simulink model "heli_q8"  (R2024b)
settings: Solver=ode1  StartTime=0.0  StopTime=inf  FixedStep=0.002  RelTol=1e-3  EnableMultiTasking=on
PostLoadFcn:
  | qc_set_target_type(getConfigSet(bdroot, 'QUARC Default Target Configuration'));
values from neighbouring files (symbols this model uses):
  A_d = 0    [kalman.m]
  B_d = 0    [kalman.m]
  C_d = 0    [kalman.m]
  Joystick_gain_x = 1    [kalman.m]
  Joystick_gain_y = -1    [kalman.m]
  Q_d = 0    [kalman.m]
  R_d = 0    [kalman.m]
  V_s0 = 0    [kalman.m]
undefined symbols (not defined in the file or in its folder): HIL, qc_get_step_size
libraries: quarc_library x4
settings Model: SimulationMode=external  ExtModeTrigDuration=5000  Creator=Rchan  LastModifiedBy=filip
settings SolverCC: AlgebraicLoopSolver=TrustRegion  PositivePriorityOrder=on
settings DataIOCC: LimitDataPoints=on  SaveFormat=Array  SignalLoggingSaveFormat=ModelDataLogs  ReturnWorkspaceOutputs=off
settings OptimizationCC: ExpressionDepthLimit=2147483647  InitFltsAndDblsToZero=on  LifeSpan=inf
settings DebuggingCC: SaveWithParameterizedLinksMsg=none  UnderspecifiedInitializationDetection=Classic  MergeDetectMultiDrivingBlocksExec=none  SolverPrmCheckMsg=warning  MultiTaskDSMMsg=warning  MultiTaskCondExecSysMsg=none  FcnCallInpInsideContextMsg=warning  UnconnectedInputMsg=warning  UnconnectedOutputMsg=warning  UnconnectedLineMsg=warning  AllowSymbolicDim=off  StateNameClashWarn=warning  SFUnexpectedBacktrackingDiag=warning  SFNoUnconditionalDefaultTransitionDiag=warning  SFExecutionAtInitializationDiag=none  ArithmeticOperatorsInVariantConditions=warning
settings HardwareCC: ProdBitPerPointer=32  ProdBitPerSizeT=32  ProdBitPerPtrDiffT=32  ProdLargestAtomicFloat=None  ProdIntDivRoundTo=Undefined  ProdEndianess=Unspecified  ProdWordSize=32  ProdHWDeviceType=32-bit Generic
settings ModelReferenceCC: EnableRefExpFcnMdlSchedulingChecks=on  PropagateSignalLabelsOutOfModel=off
settings SFSimCC: SimUseLocalCustomCode=off  CustomCodeUndefinedFunction=UseInterfaceOnly
settings RTWCC: Description=QUARC Win64 Target  SystemTargetFile=quarc_win64.tlc  TemplateMakefile=quarc_default_tmf  RTWUseLocalCustomCode=off  GPUComputeCapability=3.5
settings CodeAppCC: StateflowObjectComments=on
settings STFCustomTargetCC: TargetPreCompLibLocation=C:\PROGRA~3\QUARC\lib\2015b\win64\release  ConcurrentExecutionCompliant=on  CPPClassGenCompliant=on  GRTInterface=on  SystemTargetFile=quarc_win64.tlc
settings GRTTargetCC: TargetPreCompLibLocation=C:\PROGRA~3\QUARC\lib\2015b\win64\release  TargetLangStandard=C89/C90 (ANSI)  ParMdlRefBuildCompliant=off  CompOptLevelCompliant=off  CombineOutputUpdateFcns=off  MatFileLogging=off  GRTInterface=on  UseToolchainInfoCompliant=off  ExtMode=on  ExtModeMexFile=quarc_comm
settings ConfigComp: CovMetricSettings=dw  CovSaveCumulativeToWorkspaceVar=on  CovSaveSingleToWorkspaceVar=on  CovExternalEMLEnable=off  CovSFcnEnable=off

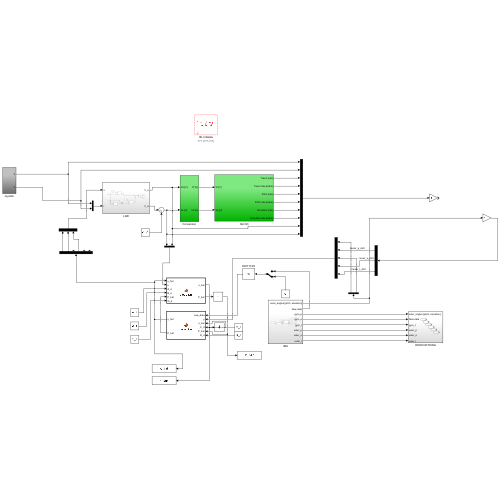
[thumbnail: Simulink's stored preview of the top-level diagram]
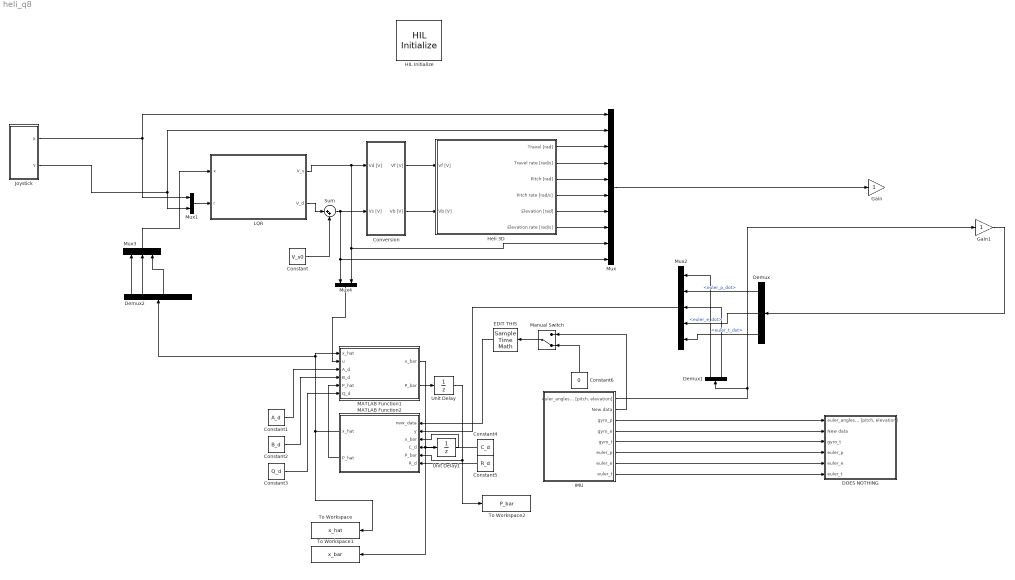
== system heli_q8 ==
  Constant : Constant  Value=V_s0
  Constant1 : Constant  Value=A_d
  Constant2 : Constant  Value=B_d
  Constant3 : Constant  Value=Q_d
  Constant4 : Constant  Value=C_d
  Constant5 : Constant  Value=R_d
  Constant6 : Constant  Value=0
  Conversion : Subsystem
  DOES NOTHING : Subsystem
  Demux : Demux  Outputs=3
  Demux1 : Demux  Outputs=2
  Demux2 : Demux  Outputs=6
  EDIT THIS : SampleTimeMath  TsampMathOp=Ts Only
  Gain : Gain
  Gain1 : Gain
  HIL Initialize : quarc_library/Data Acquisition/Generic/Configuration/HIL Initialize  Priority=-99  object_name=HIL-1  board_type=q8_usb  board_number=0  board_options=update_rate=normal;decimation=1  exclusive=off  active=off  hardware_clocks=[0:2]  clock_modes=[]  initial_clock_frequencies=[]  set_clock_params_at_start=off  set_clock_params_at_switch_in=off  set_clock_frequencies_at_start=off  set_clock_frequencies_at_switch_in=off  analog_input_channels=[0:7]  analog_input_maximums=10  analog_input_minimums=-10  set_analog_input_params_at_start=on  set_analog_input_params_at_switch_in=off  analog_output_channels=[0:7]  analog_output_maximums=10  analog_output_minimums=-10  initial_analog_outputs=[0]  final_analog_outputs=[0]  watchdog_analog_outputs=0  set_analog_output_params_at_start=on  set_analog_output_params_at_switch_in=off  set_analog_outputs_at_start=on  set_analog_outputs_at_switch_in=off  set_analog_outputs_at_terminate=on  set_analog_outputs_at_switch_out=off  set_analog_outputs_on_watchdog=off  digital_input_channels=[]  digital_output_channels=[]  digital_output_configuration=[]  initial_digital_outputs=[1]  final_digital_outputs=[1]  watchdog_digital_outputs=[1]  set_digital_output_params_at_start=off  set_digital_output_params_at_switch_in=off  set_digital_outputs_at_start=on  set_digital_outputs_at_switch_in=off  set_digital_outputs_at_terminate=on  set_digital_outputs_at_switch_out=off  set_digital_outputs_on_watchdog=off  encoder_channels=[0:7]  quadrature=[4]  encoder_filter_frequency=[]  initial_encoder_counts=[0]  set_encoder_params_at_start=on  set_encoder_params_at_switch_in=off  set_encoder_counts_at_start=on  set_encoder_counts_at_switch_in=off  pwm_channels=[0:7]  pwm_modes=0  pwm_frequency=99.532799999999995e6/4095  pwm_configuration=[0]  pwm_alignment=[0]  pwm_polarity=[1]  pwm_leading_deadband=[0]  pwm_trailing_deadband=[0]  initial_pwm_outputs=[0]  final_pwm_outputs=[0]  watchdog_pwm_outputs=[0]  set_pwm_params_at_start=on  set_pwm_params_at_switch_in=off  set_pwm_outputs_at_start=on  set_pwm_outputs_at_switch_in=off  set_pwm_outputs_at_terminate=on  set_pwm_outputs_at_switch_out=off  set_pwm_outputs_on_watchdog=off  other_output_channels=[]  initial_other_outputs=[]  final_other_outputs=[]  watchdog_other_outputs=[]  set_other_outputs_at_start=off  set_other_outputs_at_switch_in=off  set_other_outputs_at_terminate=off  set_other_outputs_at_switch_out=off  set_other_outputs_on_watchdog=off
  Heli 3D : Subsystem
  IMU : Subsystem
  Joystick : Subsystem
  LQR : Subsystem
  MATLAB Function1 : MATLAB Function  TreatAsAtomicUnit=on
  MATLAB Function2 : MATLAB Function  TreatAsAtomicUnit=on
  Manual Switch : ManualSwitch  CurrentSetting=0
  Mux : Mux  Inputs=10
  Mux1 : Mux  Inputs=2
  Mux2 : Mux  Inputs=5
  Mux3 : Mux  Inputs=3
  Mux4 : Mux  Inputs=2
  Sum : Sum  Inputs=|++
  To Workspace : ToWorkspace  VariableName=x_hat  SaveFormat=Timeseries  SampleTime=-1
  To Workspace1 : ToWorkspace  VariableName=x_bar  SaveFormat=Timeseries  SampleTime=-1
  To Workspace2 : ToWorkspace  VariableName=P_bar  SaveFormat=Timeseries  SampleTime=-1
  Unit Delay : UnitDelay  SampleTime=-1  HasFrameUpgradeWarning=on
  Unit Delay1 : UnitDelay  SampleTime=-1  HasFrameUpgradeWarning=on
  wires:
  Conversion/2(Vb [V]) -> Heli 3D/2(Vb [V])
  Conversion/1(Vf [V]) -> Heli 3D/1(Vf [V])
  Mux1/1 -> LQR/2(r)
  Joystick/1(X) -> Mux1/1, Mux/1
  Joystick/2(Y) -> Mux/2, Mux1/2
  Heli 3D/1(Travel [rad]) -> Mux/3
  Heli 3D/2(Travel rate [rad/s]) -> Mux/4
  Heli 3D/3(Pitch [rad]) -> Mux/5
  Heli 3D/4(Pitch rate [rad/s]) -> Mux/6
  Heli 3D/5(Elevation [rad]) -> Mux/7
  Heli 3D/6(Elevation rate [rad/s]) -> Mux/8
  LQR/1(V_s) -> Mux/9, Mux4/2, Conversion/1(Vd [V])
  LQR/2(V_d) -> Sum/1
  Constant/1 -> Sum/2
  Sum/1 -> Mux/10, Mux4/1, Conversion/2(Vs [V])
  Constant3/1 -> MATLAB Function1/6(Q_d)
  Constant2/1 -> MATLAB Function1/4(B_d)
  Constant1/1 -> MATLAB Function1/3(A_d)
  MATLAB Function2/2(P_hat) -> MATLAB Function1/5(P_hat)
  MATLAB Function2/1(x_hat) -> MATLAB Function1/1(x_hat), Demux2/1, To Workspace/1
  MATLAB Function1/1(x_bar) -> Unit Delay1/1, To Workspace1/1
  MATLAB Function1/2(P_bar) -> Unit Delay/1
  Unit Delay1/1 -> MATLAB Function2/3(x_bar)
  Unit Delay/1 -> To Workspace2/1, MATLAB Function2/5(P_bar)
  IMU/3(gyro_p) -> DOES NOTHING/1("euler_angles [pitch, elevation]")
  IMU/4(gyro_e) -> DOES NOTHING/2(New data)
  IMU/5(gyro_t) -> DOES NOTHING/3(gyro_t)
  IMU/6(euler_p) -> DOES NOTHING/4(euler_p)
  IMU/7(euler_e) -> DOES NOTHING/5(euler_e)
  IMU/8(euler_t) -> DOES NOTHING/6(euler_t)
  Mux/1 -> Gain/1
  IMU/1("euler_angles [pitch, elevation]") -> Demux1/1, Gain1/1
  Gain1/1 -> Demux/1
  Demux/3 -> Mux2/5  "<euler_t_dot>"
  Demux/2 -> Mux2/4  "<euler_e_dot>"
  Demux1/1 -> Mux2/1
  Demux1/2 -> Mux2/3
  Mux2/1 -> MATLAB Function2/2(y)
  Constant4/1 -> MATLAB Function2/4(C_d)
  Constant5/1 -> MATLAB Function2/6(R_d)
  Demux/1 -> Mux2/2  "<euler_p_dot>"
  EDIT THIS/1 -> MATLAB Function2/1(new_data)
  Manual Switch/1 -> EDIT THIS/1
  Constant6/1 -> Manual Switch/2
  IMU/2(New data) -> Manual Switch/1
  Demux2/1 -> Mux3/1
  Demux2/2 -> Mux3/2
  Demux2/4 -> Mux3/3
  Mux3/1 -> LQR/1(x)
  Mux4/1 -> MATLAB Function1/2(u)

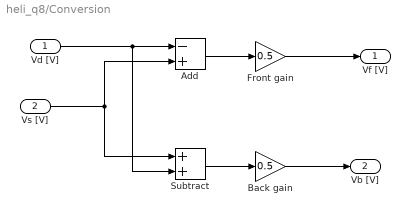
== system heli_q8/Conversion ==
  Vd [V] : Inport
  Vs [V] : Inport  Port=2
  Add : Sum  Inputs=-+
  Back gain : Gain  Gain=0.5
  Front gain : Gain  Gain=0.5
  Subtract : Sum
  Vf [V] : Outport
  Vb [V] : Outport  Port=2
  wires:
  Vd [V]/1 -> Subtract/2, Add/1
  Vs [V]/1 -> Subtract/1, Add/2
  Subtract/1 -> Back gain/1
  Back gain/1 -> Vb [V]/1
  Add/1 -> Front gain/1
  Front gain/1 -> Vf [V]/1

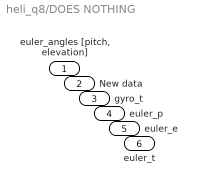
== system heli_q8/DOES NOTHING ==
  "euler_angles [pitch, elevation]" : Inport
  New data : Inport  Port=2
  gyro_t : Inport  Port=3
  euler_p : Inport  Port=4
  euler_e : Inport  Port=5
  euler_t : Inport  Port=6

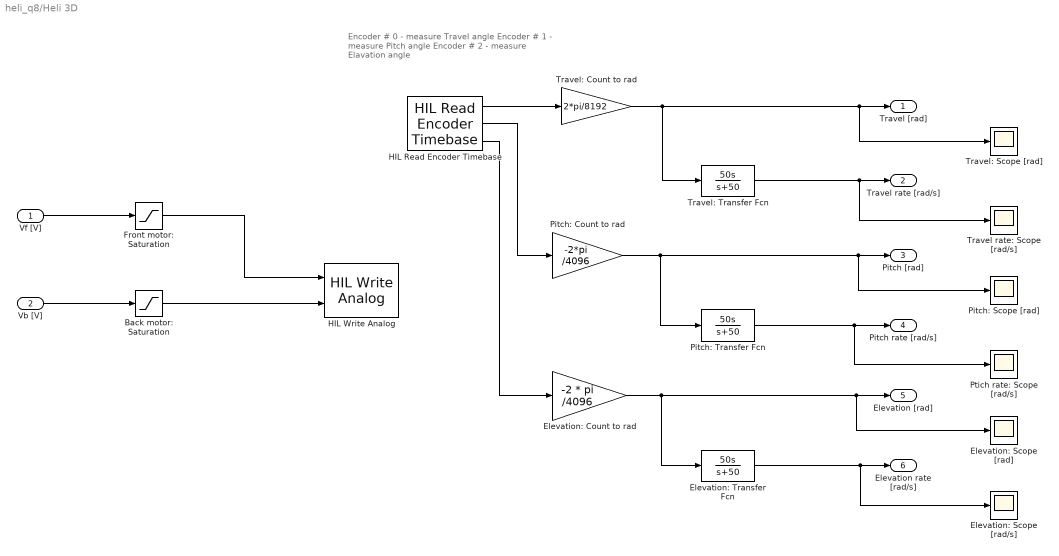
== system heli_q8/Heli 3D ==
  note: Encoder # 0 - measure Travel angle
      | Encoder # 1 - measure Pitch angle
      | Encoder # 2 - measure Elavation angle
  Vf [V] : Inport
  Vb [V] : Inport  Port=2
  Back motor: Saturation : Saturate  UpperLimit=5  LowerLimit=-5
  Elevation: Count to rad : Gain  Gain=-2 * pi /4096
  Elevation: Scope [rad/s] : Scope
  Elevation: Scope [rad] : Scope
  Elevation: Transfer Fcn : TransferFcn  Numerator=[50 0]  Denominator=[1 50]
  Front motor: Saturation : Saturate  UpperLimit=5  LowerLimit=-5
  HIL Read Encoder Timebase : quarc_library/Data Acquisition/Generic/Timebases/HIL Read Encoder Timebase  object_name=HIL-1  clock=0  channels=[0:2]  samples_in_buffer=max(ceil(1/qc_get_step_size), 1)  active=on  vector_output=off  data_type_mode=Inherit via back propagation  data_type=double
  HIL Write Analog : quarc_library/Data Acquisition/Generic/Immediate I//O/HIL Write Analog  object_name=HIL-1  channels=[0:1]  sample_time=-1  active=off  vector_input=off
  Pitch: Count to rad : Gain  Gain=-2*pi /4096
  Pitch: Scope [rad] : Scope
  Pitch: Transfer Fcn : TransferFcn  Numerator=[50 0]  Denominator=[1 50]
  Ptich rate: Scope [rad/s] : Scope
  Travel rate: Scope [rad/s] : Scope
  Travel: Count to rad : Gain  Gain=2*pi/8192
  Travel: Scope [rad] : Scope
  Travel: Transfer Fcn : TransferFcn  Numerator=[50 0]  Denominator=[1 50]
  Travel [rad] : Outport
  Travel rate [rad/s] : Outport  Port=2
  Pitch [rad] : Outport  Port=3
  Pitch rate [rad/s] : Outport  Port=4
  Elevation [rad] : Outport  Port=5
  Elevation rate [rad/s] : Outport  Port=6
  wires:
  HIL Read Encoder Timebase/1 -> Travel: Count to rad/1
  HIL Read Encoder Timebase/2 -> Pitch: Count to rad/1
  HIL Read Encoder Timebase/3 -> Elevation: Count to rad/1
  Travel: Count to rad/1 -> Travel: Scope [rad]/1, Travel [rad]/1, Travel: Transfer Fcn/1
  Travel: Transfer Fcn/1 -> Travel rate: Scope [rad/s]/1, Travel rate [rad/s]/1
  Pitch: Count to rad/1 -> Pitch: Transfer Fcn/1, Pitch: Scope [rad]/1, Pitch [rad]/1
  Pitch: Transfer Fcn/1 -> Ptich rate: Scope [rad/s]/1, Pitch rate [rad/s]/1
  Elevation: Count to rad/1 -> Elevation: Transfer Fcn/1, Elevation: Scope [rad]/1, Elevation [rad]/1
  Elevation: Transfer Fcn/1 -> Elevation: Scope [rad/s]/1, Elevation rate [rad/s]/1
  Vf [V]/1 -> Front motor: Saturation/1
  Vb [V]/1 -> Back motor: Saturation/1
  Front motor: Saturation/1 -> HIL Write Analog/1
  Back motor: Saturation/1 -> HIL Write Analog/2

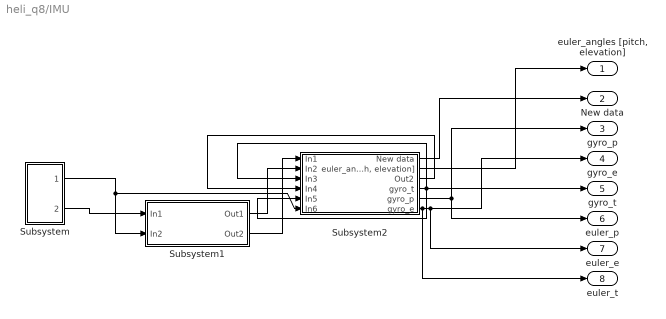
== system heli_q8/IMU ==
  Subsystem : Subsystem
  Subsystem1 : Subsystem
  Subsystem2 : Subsystem
  "euler_angles [pitch, elevation]" : Outport
  New data : Outport  Port=2
  gyro_p : Outport  Port=3
  gyro_e : Outport  Port=4
  gyro_t : Outport  Port=5
  euler_p : Outport  Port=6
  euler_e : Outport  Port=7
  euler_t : Outport  Port=8
  wires:
  Subsystem/1(Out1) -> Subsystem1/2(In2), Subsystem2/6(In6)
  Subsystem/2(Out2) -> Subsystem1/1(In1)
  Subsystem1/1(Out1) -> Subsystem2/2(In2)
  Subsystem1/2(Out2) -> Subsystem2/1(In1)
  Subsystem2/4(gyro_t) -> gyro_t/1, Subsystem2/5(In5), Subsystem2/3(In3)
  Subsystem2/3(Out2) -> Subsystem2/4(In4)
  Subsystem2/2("euler_angles [pitch, elevation]") -> "euler_angles [pitch, elevation]"/1
  Subsystem2/1(New data) -> New data/1
  Subsystem2/5(gyro_p) -> euler_p/1, gyro_p/1
  Subsystem2/6(gyro_e) -> euler_t/1, euler_e/1, gyro_e/1

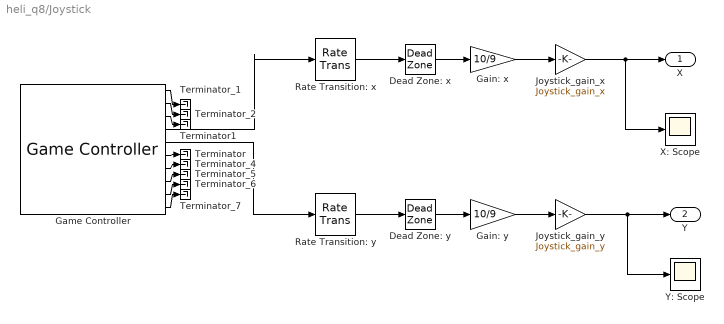
== system heli_q8/Joystick ==
  Dead Zone: x : DeadZone  LowerValue=-0.1  UpperValue=0.1
  Dead Zone: y : DeadZone  LowerValue=-0.1  UpperValue=0.1
  Gain: x : Gain  Gain=10/9
  Gain: y : Gain  Gain=10/9
  Game Controller : quarc_library/Devices/Peripherals/Target/Game Controller  controller=1  buffer_size=12  deadzone=[]  saturation=[]  sample_time=max(qc_get_step_size, 0.01)  auto_center=off  enabled=on
  Joystick_gain_x : Gain  Gain=Joystick_gain_x
  Joystick_gain_y : Gain  Gain=Joystick_gain_y
  Rate Transition: x : RateTransition
  Rate Transition: y : RateTransition
  Terminator : Terminator
  Terminator1 : Terminator
  Terminator_{1..2,4..7} (6 alike) : Terminator
  X: Scope : Scope
  Y: Scope : Scope
  X : Outport
  Y : Outport  Port=2
  wires:
  Rate Transition: y/1 -> Dead Zone: y/1
  Rate Transition: x/1 -> Dead Zone: x/1
  Game Controller/5 -> Rate Transition: y/1
  Game Controller/4 -> Rate Transition: x/1
  Game Controller/1 -> Terminator_1/1
  Game Controller/2 -> Terminator_2/1
  Game Controller/7 -> Terminator_4/1
  Game Controller/8 -> Terminator_5/1
  Game Controller/9 -> Terminator_6/1
  Game Controller/10 -> Terminator_7/1
  Game Controller/3 -> Terminator1/1
  Game Controller/6 -> Terminator/1
  Dead Zone: x/1 -> Gain: x/1
  Dead Zone: y/1 -> Gain: y/1
  Gain: x/1 -> Joystick_gain_x/1
  Gain: y/1 -> Joystick_gain_y/1
  Joystick_gain_x/1 -> X/1, X: Scope/1
  Joystick_gain_y/1 -> Y: Scope/1, Y/1

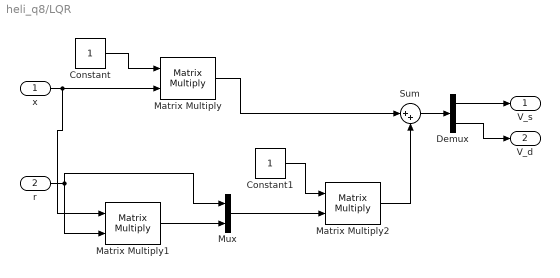
== system heli_q8/LQR ==
  x : Inport
  r : Inport  Port=2
  Constant : Constant
  Constant1 : Constant
  Demux : Demux  Outputs=2
  Matrix Multiply : Product  Multiplication=Matrix(*)
  Matrix Multiply1 : Product  Multiplication=Matrix(*)
  Matrix Multiply2 : Product  Multiplication=Matrix(*)
  Mux : Mux  Inputs=2
  Sum : Sum  Inputs=|++
  V_s : Outport
  V_d : Outport  Port=2
  wires:
  Demux/1 -> V_s/1
  Demux/2 -> V_d/1
  Sum/1 -> Demux/1
  x/1 -> Matrix Multiply1/1, Matrix Multiply/2
  Constant/1 -> Matrix Multiply/1
  Matrix Multiply/1 -> Sum/1
  r/1 -> Mux/1, Matrix Multiply1/2
  Matrix Multiply1/1 -> Mux/2
  Constant1/1 -> Matrix Multiply2/1
  Mux/1 -> Matrix Multiply2/2
  Matrix Multiply2/1 -> Sum/2

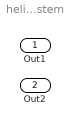
== system heli_q8/IMU/Subsystem ==
  Out1 : Outport
  Out2 : Outport  Port=2

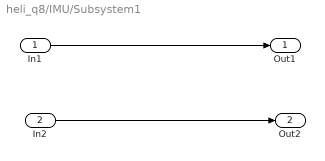
== system heli_q8/IMU/Subsystem1 ==
  In1 : Inport
  In2 : Inport  Port=2
  Out1 : Outport
  Out2 : Outport  Port=2
  wires:
  In1/1 -> Out1/1
  In2/1 -> Out2/1

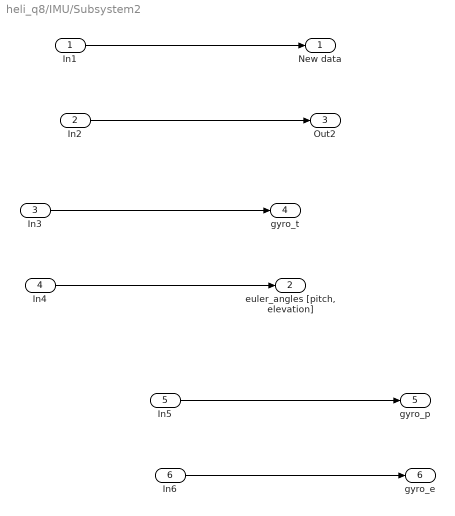
== system heli_q8/IMU/Subsystem2 ==
  In1 : Inport
  In2 : Inport  Port=2
  In3 : Inport  Port=3
  In4 : Inport  Port=4
  In5 : Inport  Port=5
  In6 : Inport  Port=6
  New data : Outport
  "euler_angles [pitch, elevation]" : Outport  Port=2
  Out2 : Outport  Port=3
  gyro_t : Outport  Port=4
  gyro_p : Outport  Port=5
  gyro_e : Outport  Port=6
  wires:
  In1/1 -> New data/1
  In2/1 -> Out2/1
  In4/1 -> "euler_angles [pitch, elevation]"/1
  In3/1 -> gyro_t/1
  In6/1 -> gyro_e/1
  In5/1 -> gyro_p/1

== matlab function heli_q8/MATLAB Function1 ==
  data: x_hat input; x_bar output; u input; A_d input; B_d input; P_hat input; Q_d input; P_bar output
function [x_bar, P_bar] = prediction(x_hat, u, A_d, B_d, P_hat, Q_d)
%#codegen
% Prediction step of a discrete-time Kalman filter
% Inputs:
%   x_hat - current state estimate
%   u     - control input
%   A_d   - discrete-time state transition matrix
%   B_d   - discrete-time control input matrix
%   P_hat - current state covariance
%   Q_d   - process noise covariance
%
% Outputs:
%   x_bar - predicted state
%   P_bar - predicted covariance

% State prediction
x_bar = A_d * x_hat + B_d * u;

% Covariance prediction
P_bar = A_d * P_hat * A_d' + Q_d;

end

== matlab function heli_q8/MATLAB Function2 ==
  data: new_data input; x_hat output; P_hat output; y input; x_bar input; C_d input; P_bar input; R_d input
function [x_hat, P_hat] =   correction(new_data, y, x_bar, C_d, P_bar, R_d)
%#codegen
% Prediction step of a discrete-time Kalman filter
% Inputs:
%   x_hat - current state estimate
%   u     - control input
%   A_d   - discrete-time state transition matrix
%   B_d   - discrete-time control input matrix
%   P_hat - current state covariance
%   Q_d   - process noise covariance
%
% Outputs:
%   x_bar - predicted state
%   P_bar - predicted covariance

% State prediction


end
